simulink model "SalientPolePMSM"  (R2020b)
settings: Solver=VariableStepAuto  StartTime=0  StopTime=1  MaxStep=1e-4  RelTol=1e-4
values from neighbouring files (symbols this model uses):
  Bgain = 1    [DataSalientPolePMSM-DESKTOP-IINSHMA.m]    (also in DataSalientPolePMSM.m)
  Gcc_1ord = 1/(s/bandwidth(Gcc) + 1)    [DataSalientPolePMSM-DESKTOP-IINSHMA.m]    (also in DataSalientPolePMSM.m)
  lamdVec = mot.Ld*idVec+mot.lammg    [DataSalientPolePMSM-DESKTOP-IINSHMA.m]    (also in DataSalientPolePMSM.m)
  lamqVec = mot.Lq*iqVec    [DataSalientPolePMSM-DESKTOP-IINSHMA.m]    (also in DataSalientPolePMSM.m)
  TAB0_abc = Tabc_AB0^-1    [DataSalientPolePMSM-DESKTOP-IINSHMA.m]    (also in DataSalientPolePMSM.m)
  Tabc_AB0 = 2/3.*[     1       -1/2       -1/2 ... (first row only)    [DataSalientPolePMSM-DESKTOP-IINSHMA.m]    (also in DataSalientPolePMSM.m)
  Talphabeta_abc = Tabc_alphabeta^(-1)    [DataSalientPolePMSM-DESKTOP-IINSHMA.m]    (also in DataSalientPolePMSM.m)
undefined symbols (not defined in the file or in its folder): DiscIntNeverNeededParam, dqpll, inv, kid, kpd, magnitude, meas, mot, Obs, PI, stconv
libraries: simulink x53, pid_lib x3, powerlib x2, eeBldcCommutationLogic x1, electricdrivelib x1
(part 7 of 7)

== matlab function SalientPolePMSM/FOC2/Circle Limitation/MATLAB Function ==
  data: u_d input; new_d output; u_q input; new_q output
function  [new_d, new_q] = Circle_limit(u_d,u_q)
if(u_d < 0)
    sign_d = -1;
else
    sign_d = 1;
end
if(u_q < 0)
    sign_q = -1;
else
    sign_q = 1;
end
    
sq_d = u_d*u_d;
sq_q = u_q*u_q;
maxModule = 31783; %PWM MAX MODELULATION 97%
sq_sum = sq_d + sq_q;
sq_limit = maxModule*maxModule;
MaxVd = (maxModule *950/1000);
sq_limit_d = MaxVd*MaxVd;
new_d = sqrt(sq_d) * sign_d;
new_q = sqrt(sq_q) * sign_q;

if(sq_sum > sq_limit)
    if (sq_d <= sq_limit_d)
        sq_tmp = sq_limit - sq_d;
        new_q = sqrt(sq_tmp);

        if (sqrt(sq_q) <= 0)
            new_q = -new_q;
        end
        new_d = sqrt(sq_d);
    else
        new_d = sq_limit_d;
        if( sqrt(sq_d) < 0)
            new_d = -new_d;
        end
        sq_tmp = sq_limit - sq_limit_d;
        new_q = sqrt(sq_tmp);
        
        if(sqrt(sq_q) < 0)
            new_q = - new_q;
        end
    end
end  

end

== matlab function SalientPolePMSM/DT SENSORLESS ALGORITHM AB/Classic PLL1/MATLAB Function2 ==
  data: u input; y output
function y = fcn(u)

if(u < 0)
    y = u * -1;
else
    y = u;
end

== matlab function SalientPolePMSM/DT SENSORLESS ALGORITHM DQ/atan ==
  data: ed input; thme output; eq input
function thme = atan(ed,eq)

thme = atan2(-ed,eq);

== matlab function SalientPolePMSM/FOC2/INVERTER1/SVM algorithm/MATLAB Function ==
  data: uABref input; sector output
function sector = sector_identifier(uABref)
% this function find the sector in the SVM where uABref is
ua = uABref(1);
ub = uABref(2);

if(ub > 0) 
    if(abs(ua) > abs(ub)/sqrt(3))
        if (ua > 0)
            sector=1;
        else
            sector=3;
        end
    else
        sector=2;
    end
else
    if(abs(ua) > abs(ub)/sqrt(3))
        if (ua > 0)
            sector=6;
        else 
            sector=4;
        end
    else
        sector=5;
    end
end

== matlab function SalientPolePMSM/FOC2/INVERTER1/SVM algorithm/MATLAB Function1 ==
  data: UABref input; uABref_sat output; uBus input; satON output
function [uABref_sat, satON] = circle_sat(UABref, uBus)
%

den = UABref(1)^2 + UABref(2)^2;
num = uBus^2/3;

if den > num
    satON = 1;
    k = sqrt(num/den);
    uABref_sat = (k.*UABref);
else
   uABref_sat = UABref; 
   satON = 0;
end

== matlab function SalientPolePMSM/INVERTER/SVM algorithm/MATLAB Function3 ==
  data: sid input; Tm_m1_0 input; uABref input; uAref_sat output; uBref_sat output; duties output; Tabc_AB0 parameter; inv parameter; satON output
function [uAref_sat, uBref_sat, duties, satON] = hexagonal_sat_sat(sid, Tm_m1_0, uABref, Tabc_AB0, inv)
%

% hexagonal saturation
if Tm_m1_0(3)<0
    satON = 1;
    k = inv.Tpwm/(Tm_m1_0(1)+Tm_m1_0(2));
    Tm_m1_0 = k.*Tm_m1_0;
    Tm_m1_0(3) = 0;
else
    satON = 0;
end

% duties calculation
duties = zeros(3,1);

switch sid
    case 1
        duties(1) = (Tm_m1_0(1)+Tm_m1_0(2)+Tm_m1_0(3)/2);
        duties(2) = (Tm_m1_0(2)+Tm_m1_0(3)/2);
        duties(3) = (Tm_m1_0(3)/2);
    case 2
        duties(1) = (Tm_m1_0(1)+Tm_m1_0(3)/2);
        duties(2) = (Tm_m1_0(1)+Tm_m1_0(2)+Tm_m1_0(3)/2);
        duties(3) = (Tm_m1_0(3)/2);
    case 3
        duties(2) = (Tm_m1_0(1)+Tm_m1_0(2)+Tm_m1_0(3)/2);
        duties(3) = (Tm_m1_0(2)+Tm_m1_0(3)/2);
        duties(1) = (Tm_m1_0(3)/2);
    case 4
        duties(3) = (Tm_m1_0(1)+Tm_m1_0(2)+Tm_m1_0(3)/2);
        duties(2) = (Tm_m1_0(1)+Tm_m1_0(3)/2);
        duties(1) = (Tm_m1_0(3)/2);
    case 5
        duties(3) = (Tm_m1_0(1)+Tm_m1_0(2)+Tm_m1_0(3)/2);
        duties(1) = (Tm_m1_0(2)+Tm_m1_0(3)/2);
        duties(2) = (Tm_m1_0(3)/2);
    case 6
        duties(1) = (Tm_m1_0(1)+Tm_m1_0(2)+Tm_m1_0(3)/2);
        duties(3) = (Tm_m1_0(1)+Tm_m1_0(3)/2);
        duties(2) = (Tm_m1_0(3)/2);
end
   duties = duties./inv.Tpwm;

% calculation of uAref_sat, uBref_sat from uABref
if Tm_m1_0(3)<=0
    H = Tabc_AB0*(duties.*inv.Ubus);
    uAref_sat = [1 0 0]*H;
    uBref_sat = [0 1 0]*H;  
else
    uAref_sat = uABref(1);
    uBref_sat = uABref(2);
end

== matlab function SalientPolePMSM/FOC2/INVERTER1/SVM algorithm/MATLAB Function2 ==
  data: sid input; Tm_m1_0 output; uABref input; uBus input; inv parameter
function Tm_m1_0 = application_time(sid, uABref, uBus, inv)
%this function calculate the application time Tm Tm+1 and T0

Tm_m1_0 = zeros(3,1);

    % PROBLEMA DI PASSAGGIO DELLA VARIABILE ALLA FUNZIONE

Tm_m1_0(1)=sqrt(3)/uBus*inv.Tpwm*(uABref(1)*inv.sector_LUT(sid,1)-uABref(2)*inv.sector_LUT(sid,2));
Tm_m1_0(2)=sqrt(3)/uBus*inv.Tpwm*(-uABref(1)*inv.sector_LUT(sid,3)+uABref(2)*inv.sector_LUT(sid,4));
Tm_m1_0(3)=inv.Tpwm-Tm_m1_0(1)-Tm_m1_0(2);

== matlab function SalientPolePMSM/Feedback1/HPF FIR4 ==
  data: thm input; wm output; meas parameter
function wm = getSpeed2(thm, meas)
% HPF FIR

persistent buffer_thm
if isempty(buffer_thm)
    buffer_thm = zeros(1,meas.enc.nTabs);
end

wm = (thm - buffer_thm(meas.enc.nTabs))/(meas.enc.nTabs*meas.enc.Ts);

for i=2:meas.enc.nTabs
    temp = buffer_thm(i);
    buffer_thm(i) = buffer_thm(1);
    buffer_thm(1) = temp;
end
buffer_thm(1) = thm;

== matlab function SalientPolePMSM/Feedback1/Hall Decoder2/Lookup table hall sensor ==
  data: thme input; Hall output
function Hall = Hall_Decoder(thme)

Hall_offset = 127; % elettrical degrees
thme = Hall_offset + thme;
k = floor(thme/(2*pi));

thme = thme - 2*k*pi;

Hall = zeros(1,5);

if ((0 <= thme) && (thme <= 60*pi/180))
    Hall(1) = 1;
    Hall(2) = 0;
    Hall(3) = 1;

elseif ((60*pi/180 < thme) && (thme <= 120*pi/180))
    Hall(1) = 1;
    Hall(2) = 0;
    Hall(3) = 0;
    
elseif ((120*pi/180 < thme) && (thme <= 180*pi/180))
    Hall(1) = 1;
    Hall(2) = 1;
    Hall(3) = 0;
    
elseif ((180*pi/180 < thme) && (thme <= 240*pi/180))
    Hall(1) = 0;
    Hall(2) = 1;
    Hall(3) = 0;
    
elseif ((240*pi/180 < thme) && (thme <= 300*pi/180))
    Hall(1) = 0;
    Hall(2) = 1;
    Hall(3) = 1;
    
elseif ((300*pi/180 < thme) && (thme <= 360*pi/180))
    Hall(1) = 0;
    Hall(2) = 0;
    Hall(3) = 1;
    
end
    
Hall(4) = bitor(bitor(Hall(1) , bitshift(Hall(2),1)) , bitshift(Hall(3),2));
Hall(5) = thme;
end

== matlab function SalientPolePMSM/Feedback1/Hall Decoder2/Update speed and angle ==
  data: Hall_state input; prev_Hall_state input; prev_wme input; thme output
function thme = Hall_Decoder(Hall_state, prev_Hall_state, prev_wme)
persistent angle;
Hall_offset = 127*pi/180;
if isempty(angle)
    angle = Hall_offset;
    thme = 0;
end

angle = prev_wme;

k = floor(angle/(2*pi));

if (Hall_state == 1) && (prev_Hall_state ~= 1)
    angle = 60*pi/180 + 2*pi*k;
    
elseif (Hall_state == 2) && (prev_Hall_state ~= 2)
    angle = 180*pi/180 + 2*pi*k;
    
elseif (Hall_state == 3) && (prev_Hall_state ~= 3)
    angle = 120*pi/180 + 2*pi*k;
        
elseif (Hall_state == 4) && (prev_Hall_state ~= 4)
    angle = 300*pi/180 + 2*pi*k;
            
elseif (Hall_state == 5) && (prev_Hall_state ~= 5)
    angle = 2*pi*k;
    
elseif (Hall_state == 6) && (prev_Hall_state ~= 6)
    angle = 240*pi/180 + 2*pi*k;                
end

thme = angle;

end

== matlab function SalientPolePMSM/Fuzzy PI1/   ==
  data: isMember_P input; isNotMember_P input; isMember output; isMember_I input; isNotMember_I input; isNotMember output
function [isMember, isNotMember] = Inference(isMember_P, isNotMember_P, isMember_I, isNotMember_I)
isMember = isMember_P + isMember_I;
isNotMember = isNotMember_P + isNotMember_I;
end

% float   compute_fuzzy_PID ( float  Err, float  AccumErr, float  Speed )
% {
%     float  isMember = 0.0;
%     float  isNotMember = 0.0;
%     evaluate_support( Err,      &P_rule, &isMember, &isNotMember );
%     evaluate_support( AccumErr, &I_rule, &isMember, &isNotMember );
%     evaluate_support( Speed,    &D_rule, &isMember, &isNotMember );
%     return  defuzzify( &O_rule, isMember, isNotMember );
% }

== matlab function SalientPolePMSM/Fuzzy PI1/    ==
  data: isMember input; tau output; isNotMember input; rule parameter
function tau = Defuzification(isMember, isNotMember, rule)

tau = (isMember * rule.O.LIMIT) + (isNotMember * -rule.O.LIMIT);

%saturation output
if  (tau > rule.O.LIMIT)  
tau = rule.O.LIMIT;
end
if  (tau < -rule.O.LIMIT)   
tau = -rule.O.LIMIT;
end
end

% float  defuzzify( rule *pRule, float isMember, float isNotMember )
% {
%     float  output;
%     output = (isMember * pRule->highlimit) + (isNotMember * pRule->lowlimit);
%     if  (output>pRule->highlimit)  output=pRule->highlimit;
%     if  (output>pRule->lowlimit)   output=pRule->lowlimit;
%     return output;
% }

== matlab function SalientPolePMSM/Fuzzy PI1/Rule base ==
  data: y output
function y = fcn()

y = 0;

== matlab function SalientPolePMSM/DT SENSORLESS ALGORITHM AB/Classic PLL1/MATLAB Function1 ==
  data: u input; y output
function y = fcn(u)

if(u < 0)
    y = u * -1;
else
    y = u;
end

== matlab function SalientPolePMSM/ 1 ==
  data: err input; rawoutput output; rule parameter
function rawoutput  = Fuzzification(err, rule)
    persistent err_acc
    if isempty(err_acc)
        err_acc =0;
    end
    %calculate accumulate error
    err_acc = err_acc + err; % I- part

    %fuzzification for proportional term
    %isMember_P = 0;
    %isNotMember_P = 0;
    
    %isMember_I = 0;
    %isNotMember_I = 0;
    
    in_value = 0;
    output = 0;
    if(err >= rule.P.LIMIT )
        in_value = rule.P.LIMIT;
    elseif( err <= -rule.P.LIMIT )
        in_value = -rule.P.LIMIT;
    end
    in_value = err;
    output = in_value * rule.P.WEIGHT;
    
    if(err_acc >= rule.I.LIMIT )
        in_value = rule.I.LIMIT;
    elseif( err_acc <= -rule.I.LIMIT )
        in_value = -rule.I.LIMIT;
    end
    in_value = err_acc;
    output = in_value * rule.I.WEIGHT + output;
    
    if(output >= rule.O.LIMIT)
        rawoutput =  rule.O.LIMIT;
    end
    if(output <= -rule.O.LIMIT)
        rawoutput =  -rule.O.LIMIT;
    else
        rawoutput = output;
    end
end

== matlab function SalientPolePMSM/DT SENSORLESS ALGORITHM AB/atan ==
  data: ed input; thme output; eq input
function thme = atan(ed,eq)

thme = atan2(-ed,eq);

== matlab function SalientPolePMSM/DT SENSORLESS ALGORITHM AB/PII/MATLAB Function1 ==
  data: u input; y output
function y = fcn(u)

if(u < 0)
    y = u * -1;
else
    y = u;
end

== matlab function SalientPolePMSM/DT SENSORLESS ALGORITHM AB/PII/MATLAB Function2 ==
  data: u input; y output
function y = fcn(u)

if(u < 0)
    y = u * -1;
else
    y = u;
end

== matlab function SalientPolePMSM/FOC2/INVERTER1/SVM algorithm/MATLAB Function3 ==
  data: sid input; Tm_m1_0 input; uABref input; uAref_sat output; uBref_sat output; duties output; Tabc_AB0 parameter; inv parameter; satON output
function [uAref_sat, uBref_sat, duties, satON] = hexagonal_sat_sat(sid, Tm_m1_0, uABref, Tabc_AB0, inv)
%

% hexagonal saturation
if Tm_m1_0(3)<0
    satON = 1;
    k = inv.Tpwm/(Tm_m1_0(1)+Tm_m1_0(2));
    Tm_m1_0 = k.*Tm_m1_0;
    Tm_m1_0(3) = 0;
else
    satON = 0;
end

% duties calculation
duties = zeros(3,1);

switch sid
    case 1
        duties(1) = (Tm_m1_0(1)+Tm_m1_0(2)+Tm_m1_0(3)/2);
        duties(2) = (Tm_m1_0(2)+Tm_m1_0(3)/2);
        duties(3) = (Tm_m1_0(3)/2);
    case 2
        duties(1) = (Tm_m1_0(1)+Tm_m1_0(3)/2);
        duties(2) = (Tm_m1_0(1)+Tm_m1_0(2)+Tm_m1_0(3)/2);
        duties(3) = (Tm_m1_0(3)/2);
    case 3
        duties(2) = (Tm_m1_0(1)+Tm_m1_0(2)+Tm_m1_0(3)/2);
        duties(3) = (Tm_m1_0(2)+Tm_m1_0(3)/2);
        duties(1) = (Tm_m1_0(3)/2);
    case 4
        duties(3) = (Tm_m1_0(1)+Tm_m1_0(2)+Tm_m1_0(3)/2);
        duties(2) = (Tm_m1_0(1)+Tm_m1_0(3)/2);
        duties(1) = (Tm_m1_0(3)/2);
    case 5
        duties(3) = (Tm_m1_0(1)+Tm_m1_0(2)+Tm_m1_0(3)/2);
        duties(1) = (Tm_m1_0(2)+Tm_m1_0(3)/2);
        duties(2) = (Tm_m1_0(3)/2);
    case 6
        duties(1) = (Tm_m1_0(1)+Tm_m1_0(2)+Tm_m1_0(3)/2);
        duties(3) = (Tm_m1_0(1)+Tm_m1_0(3)/2);
        duties(2) = (Tm_m1_0(3)/2);
end
   duties = duties./inv.Tpwm;

% calculation of uAref_sat, uBref_sat from uABref
if Tm_m1_0(3)<=0
    H = Tabc_AB0*(duties.*inv.Ubus);
    uAref_sat = [1 0 0]*H;
    uBref_sat = [0 1 0]*H;  
else
    uAref_sat = uABref(1);
    uBref_sat = uABref(2);
end

== matlab function SalientPolePMSM/FOC2/INVERTER2/SVM algorithm/MATLAB Function ==
  data: XYZ input; sector output; duty output
function [sector,duty] = sector_identifier(XYZ)
% this function find the sector in the SVM where uABref is
PWMperiod = 1/16000;

X = XYZ(1);
Y = XYZ(2);
Z = XYZ(3);

TimePhA = 0;
TimePhB = 0; 
TimePhC = 0;

if(Y < 0) 
    if(Z < 0) 
        sector = 5;
        TimePhA = (PWMperiod/2) + (Y - Z)/2;
        TimePhB = TimePhA + Z;
        TimePhC = TimePhA - Y;
    else
        if( X <= 0)
            sector = 4
            TimePhA = (PWMperiod/2) + (X - Z)/2;
            TimePhB = TimePhA + Z;
            TimePhC = TimePhB - X;
        else
            sector = 3;
            TimePhA = (PWMperiod/2) + (Y - X) /2;
            TimePhC = TimePhA - Y;
            TimePhB = TimePhC + X;
        end
    end
else
    if(Z>=0)
        sector = 2;
        TimePhA = (PWMperiod/2) + (Y - Z)/2;
        TimePhB = TimePhA + Z;
        TimePhC = TimePhA - Y;
    else
        if (X<=0)
            sector = 6;
            TimePhA = (PWMperiod/2) + (Y - X) /2;
            TimePhC = TimePhA - Y;
            TimePhB = TimePhC + X;
        else
            sector = 1;
            TimePhA = (PWMperiod/2) + (X - Z)/2;
            TimePhB = TimePhA + Z;
            TimePhC = TimePhB - X;
        end
    end
end

duty = [TimePhA*16000, TimePhB*16000, TimePhC*16000];
end

== matlab function SalientPolePMSM/FOC2/INVERTER2/SVM algorithm/MATLAB Function1 ==
  data: VABref input; X output; Y output; Z output
function [X,Y,Z] = AB2XYZ(VABref)
% this function find the sector in the SVM where uABref is

PWM_period = 5250;
Valpha = VABref(1);
Vbeta = VABref(2);

Ualpha = Valpha * sqrt(3) * PWM_period * 2;
Ubeta = -(Vbeta * PWM_period)* 2;

X = Ubeta;
Y = (Ubeta + Ualpha)/2;
Z = (Ubeta - Ualpha) / 2;
end

== matlab function SalientPolePMSM/FOC2/INVERTER2/SVM algorithm/MATLAB Function2 ==
  data: XYZ input; sector output; duty output
function [sector,duty] = sector_identifier(XYZ)
% this function find the sector in the SVM where uABref is
PWMperiod = 5250;

X = XYZ(1);
Y = XYZ(2);
Z = XYZ(3);

TimePhA = 0;
TimePhB = 0; 
TimePhC = 0;

if(Y < 0) 
    if(Z < 0) 
        sector = 5;
        TimePhA = (PWMperiod/4) + (Y - Z)/262144;
        TimePhB = TimePhA + Z/131072;
        TimePhC = TimePhA - Y/131072;
    else
        if( X <= 0)
            sector = 4;
            TimePhA = (PWMperiod/4) + (X - Z)/262144;
            TimePhB = TimePhA + Z/131072;
            TimePhC = TimePhB - X/131072;
        else
            sector = 3;
            TimePhA = (PWMperiod/4) + (Y - X) /262144;
            TimePhC = TimePhA - Y/131072;
            TimePhB = TimePhC + X/131072;
        end
    end
else
    if(Z>=0)
        sector = 2;
        TimePhA = (PWMperiod/4) + (Y - Z)/262144;
        TimePhB = TimePhA + Z/131072;
        TimePhC = TimePhA - Y/131072;
    else
        if (X<=0)
            sector = 6;
            TimePhA = (PWMperiod/4) + (Y - X) /262144;
            TimePhC = TimePhA - Y/131072;
            TimePhB = TimePhC + X/131072;
        else
            sector = 1;
            TimePhA = (PWMperiod/4) + (X - Z)/262144;
            TimePhB = TimePhA + Z/131072;
            TimePhC = TimePhB - X/131072;
        end
    end
end

duty = [2*TimePhA/5250, 2*TimePhB/5250, 2*TimePhC/5250];
end

== matlab function SalientPolePMSM/Avarage Derivative ==
  data: thm input; wm output; inv parameter
function wm = getSpeed1(thm, inv)
% avarage derivative

persistent buffer_thm
if isempty(buffer_thm)
    buffer_thm = zeros(1,11);
end

coeff = [0.0151515151500000 0.0185185185200000 0.0238095238100000 ...
0.0333333333300000 0.0555555555600000 0.1666666667 ...
-0.166666666700000 -0.0555555555600000 -0.0333333333300000 ...
-0.0238095238100000 -0.0185185185200000 -0.0151515151500000];
sum = coeff(1)*thm;
for i=2:12
    sum = sum + coeff(i)*buffer_thm(i-1);
end
wm = sum/inv.Tpwm;

for i=2:11
    temp = buffer_thm(i);
    buffer_thm(i) = buffer_thm(1);
    buffer_thm(1) = temp;
end
buffer_thm(1) = thm;

== matlab function SalientPolePMSM/FOC2/INVERTER2/SVM algorithm/MATLAB Function4 ==
  data: VABref input; X output; Y output; Z output
function [X,Y,Z] = AB2XYZ(VABref)
% this function find the sector in the SVM where uABref is

PWM_period = 1/16000;
Valpha = VABref(1);
Vbeta = VABref(2);

Ualpha = Valpha * sqrt(3) * PWM_period;
Ubeta = -(Vbeta * PWM_period);

X = Ubeta;
Y = (Ubeta + Ualpha)/2;
Z = (Ubeta - Ualpha) / 2;
end

== matlab function SalientPolePMSM/FOC2/MATLAB Function ==
  data: sens input; vdout output size=1 [0..3000]; v input; speed input; vqout output size=1 [0..3000]
function [vdout,vqout] = startup(sens,v,speed)
persistent vq;
if isempty(vq)
    vq =0;
end
if(sens == 0)
    vq = vq + 0.00001;
    vqout = 0.5;
    vdout = 0;
else
    vqout = v(2);
    vdout = v(1);
end

if(speed > 60*5)
    sens = 0;
end

== matlab function SalientPolePMSM/FOC2/PI_curr1/MATLAB Function1 ==
  settings: updateMethod=DISCRETE  sampleTime=inv.Ts
  data: u input; y output; inv parameter; kid parameter; kpd parameter
function y = PI_iq(u,inv, kid, kpd)
persistent err_int
if isempty(err_int)
    err_int =0;
end

kpd = 0.125;
kid = 0.00781;
y_prop = kpd*u; % P- part
err_int = err_int + kid*u; % I- part

% limit the integral
if err_int > inv.U_lim
    err_int = inv.U_lim;
end
if err_int < -inv.U_lim
    err_int = -inv.U_lim;
end

% compute the output voltage reference
y = y_prop + err_int;

% limit the PI output
if y > inv.U_lim
    y = inv.U_lim;
end
if y < -inv.U_lim
    y = -inv.U_lim;
end

end

== matlab function SalientPolePMSM/FOC2/PI_curr1/MATLAB Function3 ==
  settings: updateMethod=DISCRETE  sampleTime=inv.Ts
  data: u input; y output; inv parameter; kid parameter; kpd parameter
function y = PI_id(u,inv,kid, kpd)
persistent err_int
if isempty(err_int)
    err_int =0;
end

kpd = 0.125;
kid = 0.00781;
y_prop = kpd*u; % P- part
err_int = err_int + kid*u; % I- part

% limit the integral
if err_int > inv.U_lim
    err_int = inv.U_lim;
end
if err_int < -inv.U_lim
    err_int = -inv.U_lim;
end

% compute the output voltage reference
y = y_prop + err_int;

% limit the PI output
if y > inv.U_lim
    y = inv.U_lim;
end
if y < -inv.U_lim
    y = -inv.U_lim;
end

end

== matlab function SalientPolePMSM/FOC2/PI_curr2/MATLAB Function1 ==
  settings: updateMethod=DISCRETE  sampleTime=inv.Ts
  data: u input; y output; inv parameter; PI parameter
function y = PI_iq(u,inv,PI)
persistent err_int
if isempty(err_int)
    err_int =0;
end

kpd = PI.cur.kpd;
kid = PI.cur.kid;
y_prop = kpd*u; % P- part
err_int = err_int + kid*u; % I- part

% limit the integral
if err_int > inv.U_lim
    err_int = inv.U_lim;
end
if err_int < -inv.U_lim
    err_int = -inv.U_lim;
end

% compute the output voltage reference
y = y_prop + err_int;

% limit the PI output
if y > inv.U_lim
    y = inv.U_lim;
end
if y < -inv.U_lim
    y = -inv.U_lim;
end

end

== matlab function SalientPolePMSM/FOC2/PI_curr2/MATLAB Function3 ==
  settings: updateMethod=DISCRETE  sampleTime=inv.Ts
  data: u input; y output; inv parameter; PI parameter
function y = PI_id(u,inv,PI)
persistent err_int
if isempty(err_int)
    err_int =0;
end
kpd = PI.cur.kpd;
kid = PI.cur.kid;
y_prop = kpd*u; % P- part
err_int = err_int + kid*u; % I- part

% limit the integral
if err_int > inv.U_lim
    err_int = inv.U_lim;
end
if err_int < -inv.U_lim
    err_int = -inv.U_lim;
end

% compute the output voltage reference
y = y_prop + err_int;

%limit the PI output
if y > inv.U_lim
    y = inv.U_lim;
end
if y < -inv.U_lim
   y = -inv.U_lim;
end

end

== matlab function SalientPolePMSM/Fuzzy PI2/  ==
  data: err input; isMember_P output; isNotMember_P output; isMember_I output; isNotMember_I output; rule parameter
function [isMember_P, isNotMember_P,isMember_I, isNotMember_I] = Fuzzification(err, rule)
    persistent err_acc
    if isempty(err_acc)
        err_acc =0;
    end
    %calculate accumulate error
    err_acc = err_acc + err; % I- part

    %fuzzification for proportional term
    isMember_P = 0;
    isNotMember_P = 0;
    
    isMember_I = 0;
    isNotMember_I = 0;
    
    if       ( err >= rule.P.LIMIT )
        in_set = 1.0;
    elseif  ( err <= -rule.P.LIMIT  )
         in_set = 0.0;
    else
         in_set = (err + rule.P.LIMIT ) /(rule.P.LIMIT + rule.P.LIMIT );
    end
         
    isMember_P    = in_set * rule.P.WEIGHT;
    isNotMember_P =  (1.0 - in_set) * rule.P.WEIGHT;
    
    %fuzzification for integral term
    if       ( err_acc >= rule.I.LIMIT )
        in_set = 1.0;
    elseif  ( err_acc <= -rule.I.LIMIT  )
         in_set = 0.0;
    else
         in_set = (err_acc + rule.I.LIMIT ) /(rule.I.LIMIT + rule.I.LIMIT );
    end
         
    isMember_I    = in_set * rule.I.WEIGHT;
    isNotMember_I =  (1.0 - in_set) * rule.I.WEIGHT;
end

% void   evaluate_support(
%     float variable, rule *pRule, float *isMember, float *isNotMember )
% {
%     float  in_set;
%     if       ( variable >= pRule->highlimit )
%         in_set = 1.0;
%     else if  ( variable <= pRule->lowlimit )
%         in_set = 0.0;
%     else
%         in_set = (variable - pRule->lowlimit) /
%                  (pRule->highlimit - pRule->lowlimit);
% }

== matlab function SalientPolePMSM/Fuzzy PI2/   ==
  data: isMember_P input; isNotMember_P input; isMember output; isMember_I input; isNotMember_I input; isNotMember output
function [isMember, isNotMember] = Inference(isMember_P, isNotMember_P, isMember_I, isNotMember_I)
isMember = isMember_P + isMember_I;
isNotMember = isNotMember_P + isNotMember_I;
end

% float   compute_fuzzy_PID ( float  Err, float  AccumErr, float  Speed )
% {
%     float  isMember = 0.0;
%     float  isNotMember = 0.0;
%     evaluate_support( Err,      &P_rule, &isMember, &isNotMember );
%     evaluate_support( AccumErr, &I_rule, &isMember, &isNotMember );
%     evaluate_support( Speed,    &D_rule, &isMember, &isNotMember );
%     return  defuzzify( &O_rule, isMember, isNotMember );
% }

== matlab function SalientPolePMSM/DER+IIR_Butterworth ==
  data: thm input; wm output; meas parameter
function wm = getSpeed3(thm, meas)
% first derivative + IIR butterworth filter (2nd order)

persistent buffer_thm buffer_wm
if isempty(buffer_thm)
    buffer_thm = [0 0 0];
end
if isempty(buffer_wm)
    buffer_wm = [0 0];
end

%{
I compute the EAD from tustin discretization of continuous IIR transfer
function multiply to first derivative discrete transfer function.

Maybe some EAD coefficients are wrong so I use ones computed from Matlab 

k = (meas.enc.Ts*meas.enc.wn)^2;
a = 4+2*sqrt(2)*meas.enc.Ts*meas.enc.wn+k;
b = 2*k-8;
c = 4-2*sqrt(2)*meas.enc.Ts*meas.enc.wn+k;
wm = (k/meas.enc.Ts*(thm+buffer_thm(1)-buffer_thm(2)-buffer_thm(3))-b*buffer_wm(1)-c*buffer_wm(2))/a;

0.02995 z^3 + 0.02995 z^2 - 0.02995 z - 0.02995
  -----------------------------------------------
    0.000125 z^3 - 0.0001818 z^2 + 7.176e-05 z
%}

wm = ((0.0299545822080925*thm+0.0299545822080925*buffer_thm(1)-0.0299545822080925*buffer_thm(2)...
    -0.0299545822080925*buffer_thm(3))+0.000181780448281448*buffer_wm(1)-7.17577393854943e-05*buffer_wm(2))/0.000125;
 
% updet buffer variables
for i=2:length(buffer_thm)
    temp = buffer_thm(i);
    buffer_thm(i) = buffer_thm(1);
    buffer_thm(1) = temp;
end
buffer_thm(1) = thm;

for i=2:length(buffer_wm)
    temp = buffer_wm(i);
    buffer_wm(i) = buffer_wm(1);
    buffer_wm(1) = temp;
end 
buffer_wm(1) = wm;

== matlab function SalientPolePMSM/Fuzzy PI2/    ==
  data: isMember input; tau output; isNotMember input; rule parameter
function tau = Defuzification(isMember, isNotMember, rule)

tau = (isMember * rule.O.LIMIT) + (isNotMember * -rule.O.LIMIT);

%saturation output
if  (tau > rule.O.LIMIT)  
tau = rule.O.LIMIT;
end
if  (tau < -rule.O.LIMIT)   
tau = -rule.O.LIMIT;
end
end

% float  defuzzify( rule *pRule, float isMember, float isNotMember )
% {
%     float  output;
%     output = (isMember * pRule->highlimit) + (isNotMember * pRule->lowlimit);
%     if  (output>pRule->highlimit)  output=pRule->highlimit;
%     if  (output>pRule->lowlimit)   output=pRule->lowlimit;
%     return output;
% }

== matlab function SalientPolePMSM/Fuzzy PI2/Rule base ==
  data: y output
function y = fcn()

y = 0;

== matlab function SalientPolePMSM/MATLAB Function6 ==
  data: OffMtpa input; id output; i_ref input; iq output; mtpa parameter
function [id, iq]= MTPA(OffMtpa, i_ref, mtpa)
% Maximum Torque Per Ampere
if (mtpa.Ld==mtpa.Lq)||OffMtpa   % MTPA for PMSM
    id = 0;
    iq = i_ref;
else  % MTPA for IPMSM motor, or Salient Pole PMSM
    id = (mtpa.lammg-sqrt(mtpa.lammg^2+8*(mtpa.Ld-mtpa.Lq)^2*i_ref^2)/(-4*(mtpa.Ld-mtpa.Lq)));
    if i_ref>0
        iq = sqrt(i_ref^2-id^2);
        
    else
        iq = -sqrt(i_ref^2-id^2);
    end    
end

== matlab function SalientPolePMSM/Synchronous motor1/SPM Motor/MATLAB Function ==
  data: u input; B output
function B = fcn(u)
if( u>199)
    B = 0.0123;
else
    B = 0.006;
end

== matlab function SalientPolePMSM/Synchronous motor1/electrical equations/MATLAB Function ==
  data: i input; y output; Id_LUT parameter
function y = Vd_error(i,Id_LUT)
y = -0.1802*exp(-1.796*i)+0.1717;

== matlab function SalientPolePMSM/Feedback2/HPF FIR4 ==
  data: thm input; wm output; meas parameter
function wm = getSpeed2(thm, meas)
% HPF FIR

persistent buffer_thm
if isempty(buffer_thm)
    buffer_thm = zeros(1,meas.enc.nTabs);
end

wm = (thm - buffer_thm(meas.enc.nTabs))/(meas.enc.nTabs*meas.enc.Ts);

for i=2:meas.enc.nTabs
    temp = buffer_thm(i);
    buffer_thm(i) = buffer_thm(1);
    buffer_thm(1) = temp;
end
buffer_thm(1) = thm;

== matlab function SalientPolePMSM/Feedback2/Hall Decoder2/Lookup table hall sensor ==
  data: thme input; Hall output
function Hall = Hall_Decoder(thme)

Hall_offset = 127; % elettrical degrees
thme = Hall_offset + thme;
k = floor(thme/(2*pi));

thme = thme - 2*k*pi;

Hall = zeros(1,5);

if ((0 <= thme) && (thme <= 60*pi/180))
    Hall(1) = 1;
    Hall(2) = 0;
    Hall(3) = 1;

elseif ((60*pi/180 < thme) && (thme <= 120*pi/180))
    Hall(1) = 1;
    Hall(2) = 0;
    Hall(3) = 0;
    
elseif ((120*pi/180 < thme) && (thme <= 180*pi/180))
    Hall(1) = 1;
    Hall(2) = 1;
    Hall(3) = 0;
    
elseif ((180*pi/180 < thme) && (thme <= 240*pi/180))
    Hall(1) = 0;
    Hall(2) = 1;
    Hall(3) = 0;
    
elseif ((240*pi/180 < thme) && (thme <= 300*pi/180))
    Hall(1) = 0;
    Hall(2) = 1;
    Hall(3) = 1;
    
elseif ((300*pi/180 < thme) && (thme <= 360*pi/180))
    Hall(1) = 0;
    Hall(2) = 0;
    Hall(3) = 1;
    
end
    
Hall(4) = bitor(bitor(Hall(1) , bitshift(Hall(2),1)) , bitshift(Hall(3),2));
Hall(5) = thme;
end

== matlab function SalientPolePMSM/Feedback2/Hall Decoder2/Update speed and angle ==
  data: Hall_state input; prev_Hall_state input; prev_wme input; thme output
function thme = Hall_Decoder(Hall_state, prev_Hall_state, prev_wme)
persistent angle;
Hall_offset = 127*pi/180;
if isempty(angle)
    angle = Hall_offset;
    thme = 0;
end

angle = prev_wme;

k = floor(angle/(2*pi));

if (Hall_state == 1) && (prev_Hall_state ~= 1)
    angle = 60*pi/180 + 2*pi*k;
    
elseif (Hall_state == 2) && (prev_Hall_state ~= 2)
    angle = 180*pi/180 + 2*pi*k;
    
elseif (Hall_state == 3) && (prev_Hall_state ~= 3)
    angle = 120*pi/180 + 2*pi*k;
        
elseif (Hall_state == 4) && (prev_Hall_state ~= 4)
    angle = 300*pi/180 + 2*pi*k;
            
elseif (Hall_state == 5) && (prev_Hall_state ~= 5)
    angle = 2*pi*k;
    
elseif (Hall_state == 6) && (prev_Hall_state ~= 6)
    angle = 240*pi/180 + 2*pi*k;                
end

thme = angle;

end

== matlab function SalientPolePMSM/HPF FIR ==
  data: thm input; wm output; meas parameter
function wm = getSpeed2(thm, meas)
% HPF FIR

persistent buffer_thm
if isempty(buffer_thm)
    buffer_thm = zeros(1,meas.enc.nTabs);
end

wm = (thm - buffer_thm(meas.enc.nTabs))/(meas.enc.nTabs*meas.enc.Ts);

for i=2:meas.enc.nTabs
    temp = buffer_thm(i);
    buffer_thm(i) = buffer_thm(1);
    buffer_thm(1) = temp;
end
buffer_thm(1) = thm;

== matlab function SalientPolePMSM/Discrete SS ALGORITHM/atanApprox ==
  data: id input; ed input; thme output; wme_est input; dqpll parameter
function thme = approx(id, ed, wme_est, dqpll)
if abs(wme_est)<dqpll.minw
    wme_est = dqpll.minw;
end
Eex = wme_est*((dqpll.Ld-dqpll.Lq)*id+dqpll.lammg);
thme = -ed/Eex;

== matlab function SalientPolePMSM/Discrete SS ALGORITHM/atan ==
  data: ed input; thme output; eq input
function thme = atan(ed,eq)

thme = atan2(-ed,eq);
